simulink subsystem "GenCtrl"  (R2022b)
settings: Solver=VariableStepAuto  StartTime=0.0  StopTime=10.0  RelTol=1e-3
settings Model: Creator=tbritton  LastModifiedBy=macheson
settings SolverCC: AlgebraicLoopSolver=TrustRegion
settings DebuggingCC: UnconnectedInputMsg=warning  UnconnectedOutputMsg=warning  UnconnectedLineMsg=warning  SFMachineParentedDataDiag=warning
settings ModelReferenceCC: EnableRefExpFcnMdlSchedulingChecks=on
settings RTWCC: DLArmComputeVersion=19.05

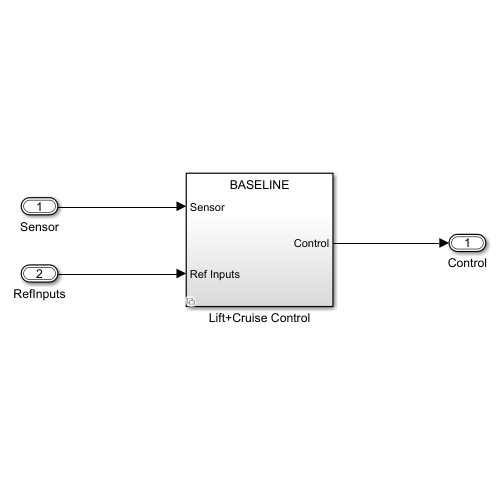
[thumbnail: Simulink's stored preview of the top-level diagram]
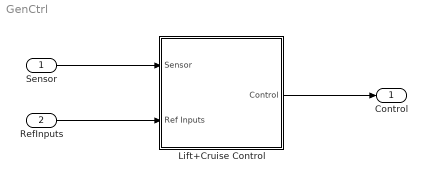
== system GenCtrl ==
  Sensor : Inport  OutDataTypeStr=Bus: SensorBus
  RefInputs : Inport  Port=2  OutDataTypeStr=Bus: BUS_REF_INPUT
  Lift+Cruise Control : Subsystem  Variant=on
  Control : Outport  OutDataTypeStr=Bus: BUS_CONTROL
  wires:
  Sensor/1 -> Lift+Cruise Control/1(Sensor)
  RefInputs/1 -> Lift+Cruise Control/2(Ref Inputs)
  Lift+Cruise Control/1(Control) -> Control/1

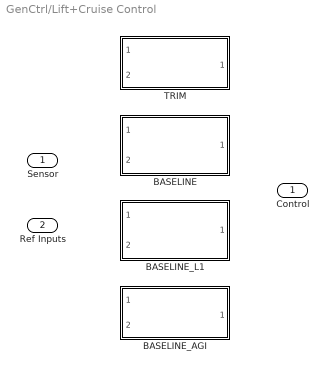
== system GenCtrl/Lift+Cruise Control ==
  Sensor : Inport  OutDataTypeStr=Bus: SensorBus
  Ref Inputs : Inport  Port=2  OutDataTypeStr=Bus: BUS_REF_INPUT
  BASELINE : Subsystem  VariantControl=GVS_CTRL_TYPE_BASELINE  ReferencedSubsystem=Baseline
  BASELINE_AGI : Subsystem  VariantControl=GVS_CTRL_TYPE_BASELINE_AGI  ReferencedSubsystem=BASELINE_AGI
  BASELINE_L1 : Subsystem  VariantControl=GVS_CTRL_TYPE_BASELINE_L1  ReferencedSubsystem=Baseline_L1
  TRIM : Subsystem  VariantControl=GVS_CTRL_TYPE_TRIM  ReferencedSubsystem=TRIM
  Control : Outport  OutDataTypeStr=Bus: BUS_CONTROL  VectorParamsAs1DForOutWhenUnconnected=off
